simulink model "MixingTank_IntegralControl_Simulink2017b"  (R2017b)
settings: Solver=ode4  StartTime=0.0  StopTime=SIM_TIME  FixedStep=STEP_SIZE  RelTol=1e-3
undefined symbols (not defined in the file): At, Cv, Kfs, kh, Ki, kt, kv, Ts, u0, x0, xi0
settings Model: Creator=Roberto  LastModifiedBy=Roberto

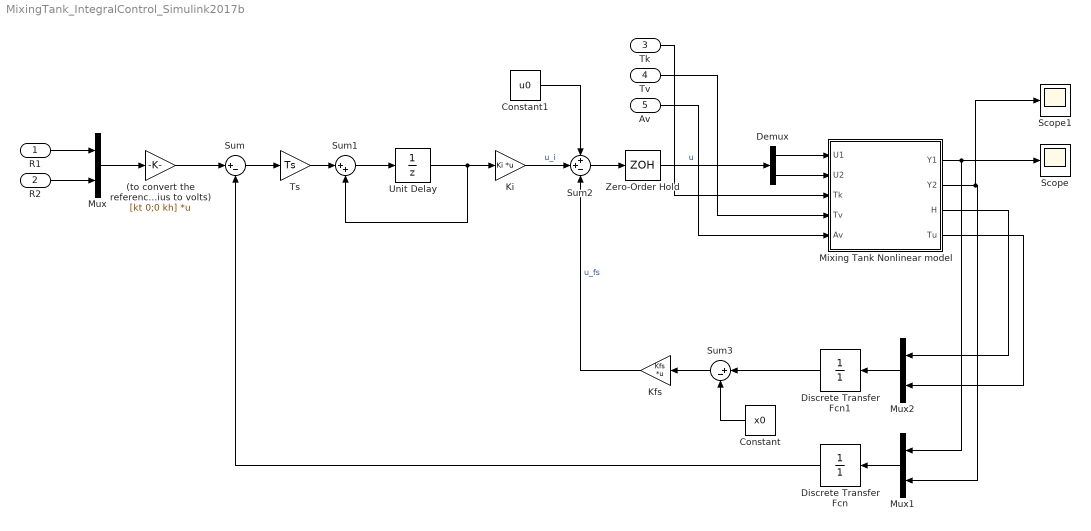
== system MixingTank_IntegralControl_Simulink2017b ==
  R1 : Inport
  R2 : Inport  Port=2
  Tk : Inport  Port=3
  Tv : Inport  Port=4
  Av : Inport  Port=5
  (to convert the reference from meters and degree Celsius to volts) : Gain  Gain=[kt 0;0 kh]  Multiplication=Matrix(K*u) (u vector)
  Constant : Constant  Value=x0
  Constant1 : Constant  Value=u0
  Demux : Demux  Outputs=2
  Discrete Transfer Fcn : DiscreteTransferFcn  Denominator=[1]  SampleTime=Ts
  Discrete Transfer Fcn1 : DiscreteTransferFcn  Denominator=[1]  SampleTime=Ts
  Kfs : Gain  Gain=Kfs  Multiplication=Matrix(K*u) (u vector)
  Ki : Gain  Gain=Ki  Multiplication=Matrix(K*u) (u vector)
  Mixing Tank Nonlinear model : Subsystem
  Mux : Mux  Inputs=2
  Mux1 : Mux  Inputs=2
  Mux2 : Mux  Inputs=2
  Scope : Scope
  Scope1 : Scope
  Sum : Sum  Inputs=|+-
  Sum1 : Sum  Inputs=|++
  Sum2 : Sum  Inputs=++-
  Sum3 : Sum  Inputs=|+-
  Ts : Gain  Gain=Ts
  Unit Delay : UnitDelay  Priority=3  InitialCondition=xi0  SampleTime=Ts
  Zero-Order Hold : ZeroOrderHold  SampleTime=Ts
  wires:
  Tk/1 -> Mixing Tank Nonlinear model/3(Tk)
  Tv/1 -> Mixing Tank Nonlinear model/4(Tv)
  Av/1 -> Mixing Tank Nonlinear model/5(Av)
  Mixing Tank Nonlinear model/1(Y1) -> Scope/1, Mux1/1
  R1/1 -> Mux/1
  R2/1 -> Mux/2
  Mux/1 -> (to convert the reference from meters and degree Celsius to volts)/1
  Sum/1 -> Ts/1
  Sum1/1 -> Unit Delay/1
  Unit Delay/1 -> Ki/1, Sum1/2
  Mux1/1 -> Discrete Transfer Fcn/1
  Discrete Transfer Fcn/1 -> Sum/2
  Ki/1 -> Sum2/2  "u_i"
  Sum2/1 -> Zero-Order Hold/1
  Kfs/1 -> Sum2/3  "u_fs"
  Demux/2 -> Mixing Tank Nonlinear model/2(U2)
  Demux/1 -> Mixing Tank Nonlinear model/1(U1)
  Zero-Order Hold/1 -> Demux/1  "u"
  Sum3/1 -> Kfs/1
  Constant/1 -> Sum3/2
  Mux2/1 -> Discrete Transfer Fcn1/1
  Mixing Tank Nonlinear model/3(H) -> Mux2/1
  Mixing Tank Nonlinear model/4(Tu) -> Mux2/2
  Constant1/1 -> Sum2/1
  Mixing Tank Nonlinear model/2(Y2) -> Scope1/1, Mux1/2
  Ts/1 -> Sum1/1
  (to convert the reference from meters and degree Celsius to volts)/1 -> Sum/1
  Discrete Transfer Fcn1/1 -> Sum3/1

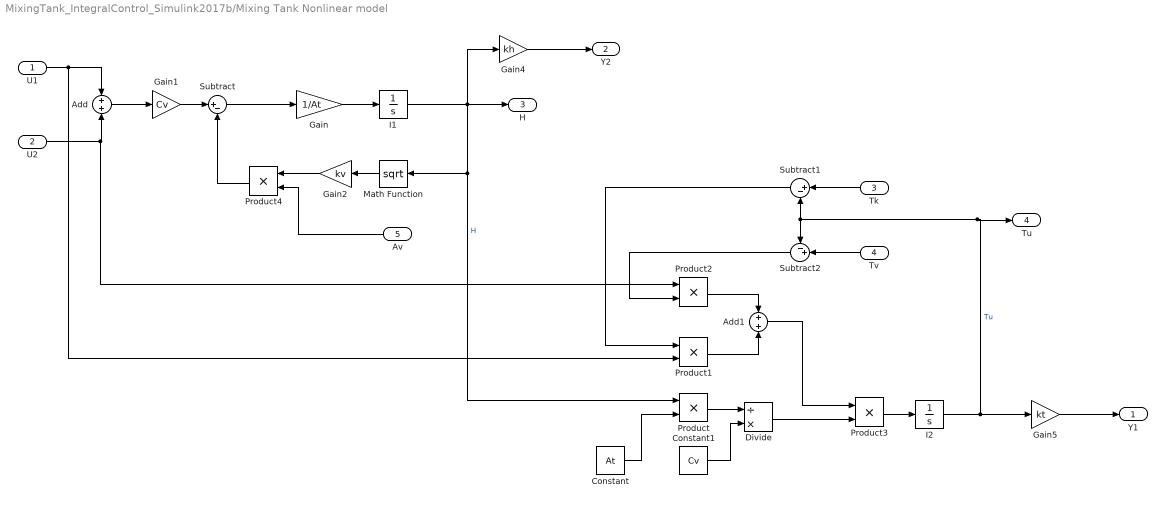
== system MixingTank_IntegralControl_Simulink2017b/Mixing Tank Nonlinear model ==
  U1 : Inport
  U2 : Inport  Port=2
  Tk : Inport  Port=3
  Tv : Inport  Port=4
  Av : Inport  Port=5
  Add : Sum
  Add1 : Sum
  Constant : Constant  Value=At
  Constant1 : Constant  Value=Cv
  Divide : Product  Inputs=/*
  Gain : Gain  Gain=1/At
  Gain1 : Gain  Gain=Cv
  Gain2 : Gain  Gain=kv
  Gain4 : Gain  Gain=kh
  Gain5 : Gain  Gain=kt
  I1 : Integrator  Priority=1  InitialCondition=x0(1)  LimitOutput=on  LowerSaturationLimit=0
  I2 : Integrator  Priority=2  InitialCondition=x0(2)
  Math Function : Math  Operator=sqrt  SaturateOnIntegerOverflow=on
  Product{,1..4} (5 alike) : Product  RndMeth=Zero
  Subtract : Sum  Inputs=|+-
  Subtract1 : Sum  Inputs=|+-
  Subtract2 : Sum  Inputs=-+|
  Y1 : Outport
  Y2 : Outport  Port=2
  H : Outport  Port=3
  Tu : Outport  Port=4
  wires:
  Math Function/1 -> Gain2/1
  Gain2/1 -> Product4/1
  Product/1 -> Divide/1
  Subtract1/1 -> Product1/1
  Product3/1 -> I2/1
  I1/1 -> H/1, Math Function/1, Product/1, Gain4/1  "H"
  Product4/1 -> Subtract/2
  Av/1 -> Product4/2
  Gain1/1 -> Subtract/1
  Add1/1 -> Product3/1
  Constant/1 -> Product/2
  Subtract2/1 -> Product2/2
  Tk/1 -> Subtract1/1
  Add/1 -> Gain1/1
  U1/1 -> Product1/2, Add/1
  Constant1/1 -> Divide/2
  Gain/1 -> I1/1
  U2/1 -> Product2/1, Add/2
  Subtract/1 -> Gain/1
  I2/1 -> Gain5/1, Tu/1, Subtract2/1, Subtract1/2  "Tu"
  Gain4/1 -> Y2/1
  Gain5/1 -> Y1/1
  Tv/1 -> Subtract2/2
  Divide/1 -> Product3/2
  Product2/1 -> Add1/1
  Product1/1 -> Add1/2
